simulink model "rfsoc_sdfec_model"  (R2020b)
settings: Solver=VariableStepAuto  StartTime=0.0  StopTime=T  RelTol=1e-3
values from neighbouring files (symbols this model uses):
  aximm_bit_count_reset = 0    [setup.m]
  aximm_bits = n_blocks * k    (= 80)    [setup.m]
  aximm_ctrl_word_dec = 0    [setup.m]
  aximm_ctrl_word_enc = 999    [setup.m]
  aximm_enable = 1    [setup.m]
  aximm_length = k * n_blocks    (= 80)    [setup.m]
  aximm_length_dec = n    (= 160)    [setup.m]
  aximm_length_enc = k/8    (= 10)    [setup.m]
  aximm_llr_scale = (1/noise_var) * llr_scale * 2    (= 200)    [setup.m]
  aximm_noise_std = sqrt(noise_var/2)    [setup.m]
  aximm_reset = 0    [setup.m]
  d = sqrt(-2*log([0:1/4095:1]))    [setup.m]
  fs = 100e6    (= 100000000)    [setup.m]
  generator_polynomial = '''z^13 + z^12 + z^11 + z^8 + 1'''    [setup.m]
libraries: hdlsllib x52, commseqgen3 x28, commblkcod2 x2, simulink x2
(part 1 of 2)
settings Model: Creator=ckb13136  LastModifiedBy=ckb13136
settings OptimizationCC: BlockReduction=off  ConditionallyExecuteInputs=off

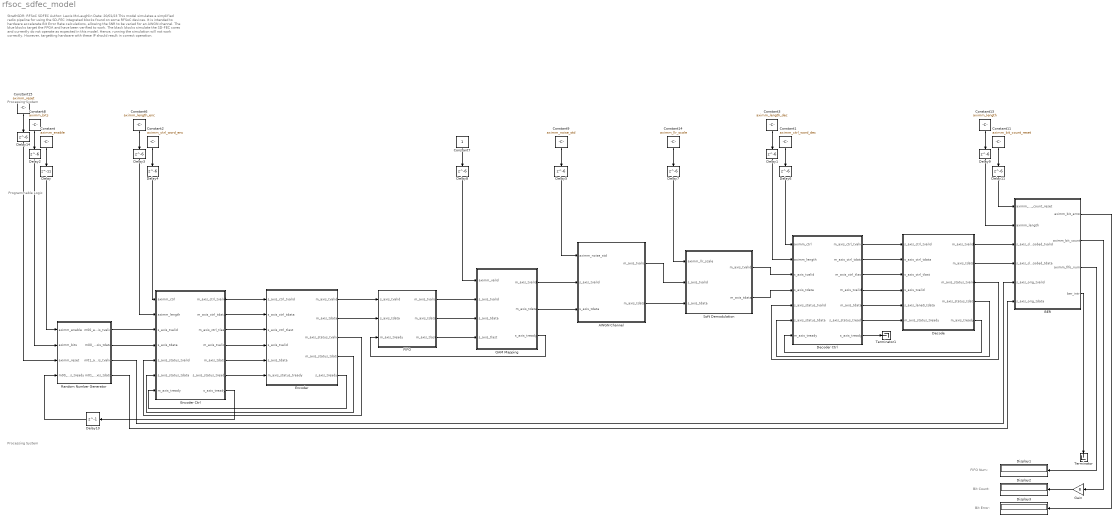
== system rfsoc_sdfec_model ==
  note: StrathSDR: RFSoC SDFEC
      | Author: Lewis McLaughlin
      | Date: 20/01/23
      |
      | This model simulates a simplified radio pipeline for using the SD-FEC integrated blocks found on some RFSoC devices. It is intended to hardware accelerate Bit Error Rate calculations, allowing the SNR to be varied for an AWGN channel. The blue blocks target the FPGA and have been verified to work. The black blocks simulate the SD-FEC cores and currently do not operate as expected in this model. Hence, running the simulation will not work correctly. However, targetting hardware with these IP should result in correct operation.
  note: FIFO Num:
  note: Programmable Logic
  note: Processing System
  note: Processing System
  note: Bit Count:
  note: Bit Error:
  AWGN Channel : Subsystem  TreatAsAtomicUnit=on
  BER : Subsystem  TreatAsAtomicUnit=on
  Constant : Constant  Value=aximm_enable  OutDataTypeStr=uint32  SampleTime=1/fs
  Constant1 : Constant  Value=aximm_ctrl_word_dec  OutDataTypeStr=uint32  SampleTime=1/fs
  Constant11 : Constant  Value=aximm_bit_count_reset  VectorParams1D=off  OutDataTypeStr=uint32  SampleTime=1/(fs)
  Constant13 : Constant  Value=aximm_length  OutDataTypeStr=uint32  SampleTime=1/(fs)
  Constant14 : Constant  Value=aximm_llr_scale  OutDataTypeStr=fixdt(0,32,12)  SampleTime=1/(fs)
  Constant15 : Constant  Value=aximm_reset  OutDataTypeStr=uint32  SampleTime=1/fs
  Constant2 : Constant  Value=aximm_ctrl_word_enc  OutDataTypeStr=uint32  SampleTime=1/fs
  Constant3 : Constant  Value=aximm_length_dec  OutDataTypeStr=uint32  SampleTime=1/fs
  Constant6 : Constant  Value=aximm_length_enc  OutDataTypeStr=uint32  SampleTime=1/fs
  Constant7 : Constant  OutDataTypeStr=uint32  SampleTime=1/fs
  Constant8 : Constant  Value=aximm_bits  OutDataTypeStr=uint32  SampleTime=1/fs
  Constant9 : Constant  Value=aximm_noise_std  OutDataTypeStr=fixdt(0,32,30)  SampleTime=1/(fs)
  Decode : Subsystem
  Decoder Ctrl : Subsystem  TreatAsAtomicUnit=on
  Delay : Delay  DelayLength=11
  Delay{1..9,11,14} (11 alike) : Delay  DelayLength=6
  Delay10 : Delay  DelayLength=1
  Display1 : Display
  Display2 : Display
  Display3 : Display
  Encoder : Subsystem
  Encoder Ctrl : Subsystem  TreatAsAtomicUnit=on
  FIFO : Subsystem
  Gain : Gain  Gain=8
  QAM Mapping : Subsystem  TreatAsAtomicUnit=on
  Random Number Generator : Subsystem  TreatAsAtomicUnit=on
  Soft Demodulation : Subsystem  TreatAsAtomicUnit=on
  Terminator : Terminator
  Terminator1 : Terminator
  wires:
  Delay/1 -> Random Number Generator/1(aximm_enable)
  Delay14/1 -> Random Number Generator/3(aximm_reset)
  Constant15/1 -> Delay14/1
  Delay2/1 -> Random Number Generator/2(aximm_bits)
  Constant/1 -> Delay/1
  Constant8/1 -> Delay2/1
  Random Number Generator/2(m00_axis_tdata) -> Encoder Ctrl/4(s_axis_tdata)
  Random Number Generator/1(m00_axis_tvalid) -> Encoder Ctrl/3(s_axis_tvalid)
  Encoder Ctrl/7(s_axis_tready) -> Delay10/1
  Encoder Ctrl/1(m_axis_ctrl_tvalid) -> Encoder/1(s_axis_ctrl_tvalid)
  Encoder Ctrl/2(m_axis_ctrl_tdata) -> Encoder/2(s_axis_ctrl_tdata)
  Encoder Ctrl/3(m_axis_ctrl_tlast) -> Encoder/3(s_axis_ctrl_tlast)
  Encoder Ctrl/4(m_axis_tvalid) -> Encoder/4(s_axis_tvalid)
  Encoder Ctrl/5(m_axis_tdata) -> Encoder/5(s_axis_tdata)
  Encoder Ctrl/6(s_axis_status_tready) -> Encoder/6(m_axis_status_tready)
  Encoder/4(m_axis_status_tdata) -> Encoder Ctrl/6(s_axis_status_tdata)
  Encoder/3(m_axis_status_tvalid) -> Encoder Ctrl/5(s_axis_status_tvalid)
  Delay4/1 -> Encoder Ctrl/1(aximm_ctrl)
  Constant2/1 -> Delay4/1
  Constant6/1 -> Delay3/1
  Delay3/1 -> Encoder Ctrl/2(aximm_length)
  Encoder/5(s_axis_tready) -> Encoder Ctrl/7(m_axis_tready)
  Encoder/1(m_axis_tvalid) -> FIFO/1(s_axis_tvalid)
  Encoder/2(m_axis_tdata) -> FIFO/2(s_axis_tdata)
  FIFO/1(m_axis_tvalid) -> QAM Mapping/2(s_axis_tvalid)
  FIFO/2(m_axis_tdata) -> QAM Mapping/3(s_axis_tdata)
  FIFO/3(m_axis_tlast) -> QAM Mapping/4(s_axis_tlast)
  QAM Mapping/3(s_axis_tready) -> FIFO/3(m_axis_tready)
  QAM Mapping/1(m_axis_tvalid) -> AWGN Channel/2(s_axis_tvalid)
  QAM Mapping/2(m_axis_tdata) -> AWGN Channel/3(s_axis_tdata)
  Constant9/1 -> Delay5/1
  Delay5/1 -> AWGN Channel/1(aximm_noise_std)
  AWGN Channel/2(m_axis_tdata) -> Soft Demodulation/3(s_axis_tdata)
  AWGN Channel/1(m_axis_tvalid) -> Soft Demodulation/2(s_axis_tvalid)
  Soft Demodulation/2(m_axis_tdata) -> Decoder Ctrl/4(s_axis_tdata)
  Soft Demodulation/1(m_axis_tvalid) -> Decoder Ctrl/3(s_axis_tvalid)
  Delay10/1 -> Random Number Generator/4(m00_axis_tready)
  Decoder Ctrl/1(m_axis_ctrl_tvalid) -> Decode/1(s_axis_ctrl_tvalid)
  Decoder Ctrl/2(m_axis_ctrl_tdata) -> Decode/2(s_axis_ctrl_tdata)
  Decoder Ctrl/3(m_axis_ctrl_tlast) -> Decode/3(s_axis_ctrl_tlast)
  Decoder Ctrl/4(m_axis_tvalid) -> Decode/4(s_axis_tvalid)
  Decoder Ctrl/5(m_axis_tdata) -> Decode/5(s_axis_lane0_tdata)
  Decoder Ctrl/6(s_axis_status_tready) -> Decode/6(m_axis_status_tready)
  Decode/5(m_axis_tready) -> Decoder Ctrl/7(m_axis_tready)
  Decode/4(m_axis_status_tdata) -> Decoder Ctrl/6(s_axis_status_tdata)
  Decode/3(m_axis_status_tvalid) -> Decoder Ctrl/5(s_axis_status_tvalid)
  Delay1/1 -> Decoder Ctrl/2(aximm_length)
  Constant3/1 -> Delay1/1
  Constant1/1 -> Delay6/1
  Delay6/1 -> Decoder Ctrl/1(aximm_ctrl)
  Constant14/1 -> Delay7/1
  Delay7/1 -> Soft Demodulation/1(aximm_llr_scale)
  Constant7/1 -> Delay8/1
  Delay8/1 -> QAM Mapping/1(aximm_valid)
  Decode/1(m_axis_tvalid) -> BER/3(s_axis_decoded_tvalid)
  Decode/2(m_axis_tdata) -> BER/4(s_axis_decoded_tdata)
  Random Number Generator/4(m01_axis_tdata) -> BER/6(s_axis_orig_tdata)
  Random Number Generator/3(m01_axis_tvalid) -> BER/5(s_axis_orig_tvalid)
  Delay11/1 -> BER/1(aximm_bit_count_reset)
  Constant11/1 -> Delay11/1
  Delay9/1 -> BER/2(aximm_length)
  Constant13/1 -> Delay9/1
  BER/4(ber_intr) -> Terminator/1
  BER/3(aximm_fifo_num) -> Display1/1
  BER/2(aximm_bit_count) -> Gain/1
  BER/1(aximm_bit_error) -> Display3/1
  Gain/1 -> Display2/1
  Decoder Ctrl/7(s_axis_tready) -> Terminator1/1

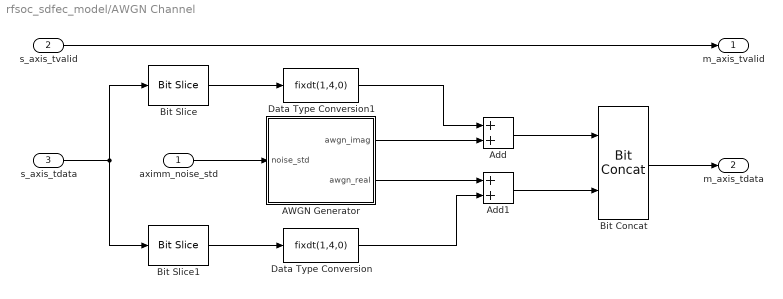
== system rfsoc_sdfec_model/AWGN Channel ==
  aximm_noise_std : Inport
  s_axis_tvalid : Inport  Port=2
  s_axis_tdata : Inport  Port=3
  AWGN Generator : Subsystem
  Add : Sum  OutDataTypeStr=fixdt(1,16,11)  SaturateOnIntegerOverflow=on
  Add1 : Sum  OutDataTypeStr=fixdt(1,16,11)  SaturateOnIntegerOverflow=on
  Bit Concat : hdlsllib/Logic and Bit Operations/Bit Concat  numInputs=2
  Bit Slice : hdlsllib/Logic and Bit Operations/Bit Slice  lidx=7  ridx=4
      settings: SourceProductBaseCode=SL
  Bit Slice1 : hdlsllib/Logic and Bit Operations/Bit Slice  lidx=3  ridx=0
      settings: SourceProductBaseCode=SL
  Data Type Conversion : DataTypeConversion  OutDataTypeStr=fixdt(1,4,0)  ConvertRealWorld=Stored Integer (SI)
  Data Type Conversion1 : DataTypeConversion  OutDataTypeStr=fixdt(1,4,0)  ConvertRealWorld=Stored Integer (SI)
  m_axis_tvalid : Outport
  m_axis_tdata : Outport  Port=2
  wires:
  Data Type Conversion1/1 -> Add/1
  Data Type Conversion/1 -> Add1/2
  Bit Slice/1 -> Data Type Conversion1/1
  Bit Slice1/1 -> Data Type Conversion/1
  s_axis_tvalid/1 -> m_axis_tvalid/1
  Bit Concat/1 -> m_axis_tdata/1
  s_axis_tdata/1 -> Bit Slice/1, Bit Slice1/1
  aximm_noise_std/1 -> AWGN Generator/1(noise_std)
  AWGN Generator/1(awgn_imag) -> Add/2
  AWGN Generator/2(awgn_real) -> Add1/1
  Add1/1 -> Bit Concat/2
  Add/1 -> Bit Concat/1

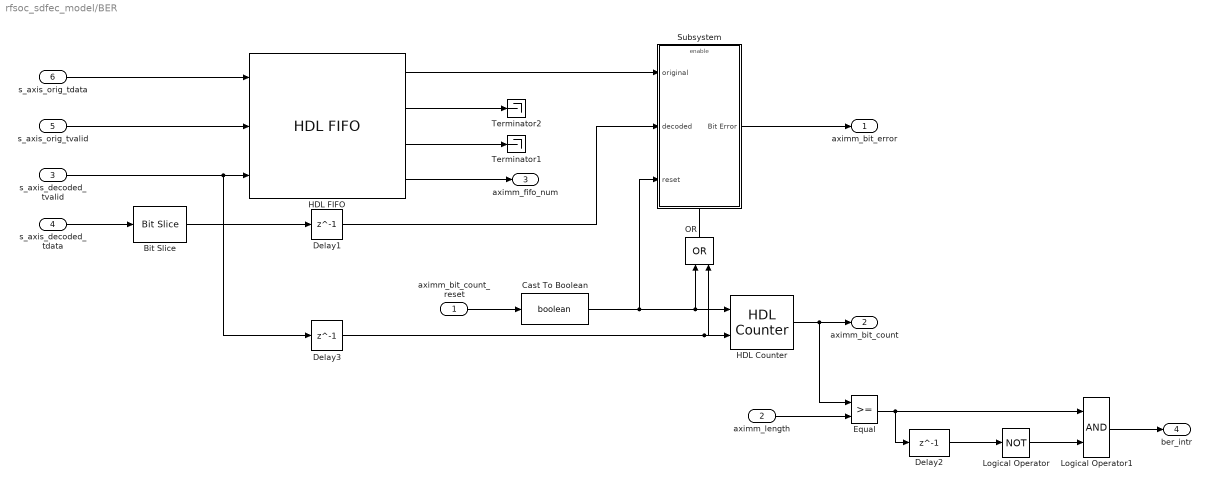
== system rfsoc_sdfec_model/BER ==
  aximm_bit_count_reset : Inport
  aximm_length : Inport  Port=2
  s_axis_decoded_tvalid : Inport  Port=3
  s_axis_decoded_tdata : Inport  Port=4
  s_axis_orig_tvalid : Inport  Port=5
  s_axis_orig_tdata : Inport  Port=6
  Bit Slice : hdlsllib/Logic and Bit Operations/Bit Slice  lidx=7  ridx=0
      settings: SourceProductBaseCode=SL
  Cast To Boolean : DataTypeConversion  OutDataTypeStr=boolean
  Delay1 : Delay  DelayLength=1
  Delay2 : Delay  DelayLength=1  InitialCondition=1  InputProcessing=Columns as channels (frame based)
  Delay3 : Delay  DelayLength=1
  Equal : RelationalOperator  OutDataTypeStr=boolean  RndMeth=Simplest
  HDL Counter : hdlsllib/Sources/HDL Counter  CountType=Free running  CountInit=0  CountStep=1  CountMax=25  CountFromType=Initial value  CountFrom=0  CountResetPort=on  CountLoadPort=off  CountEnbPort=on  CountDirPort=off  CountDataType=Unsigned  CountWordLen=32  CountFracLen=0  CountSampTime=1
  HDL FIFO : hdlsllib/HDL RAMs/HDL FIFO  fifo_size=65536  mode=Classic  ratio=1  push_msg=Warning  pop_msg=Warning  show_empty=on  show_full=on  show_num=on  LabelModeActiveChoice_Mode=Classic
      settings: SourceProductBaseCode=SL
  Logical Operator : Logic  Operator=NOT  Inputs=1
  Logical Operator1 : Logic
  OR : Logic  Operator=OR  IconShape=distinctive  AllPortsSameDT=off  OutDataTypeStr=boolean
  Subsystem : Subsystem
  Terminator1 : Terminator
  Terminator2 : Terminator
  aximm_bit_error : Outport
  aximm_bit_count : Outport  Port=2
  aximm_fifo_num : Outport  Port=3
  ber_intr : Outport  Port=4
  wires:
  HDL FIFO/4 -> aximm_fifo_num/1
  s_axis_decoded_tvalid/1 -> HDL FIFO/3, Delay3/1
  Delay3/1 -> OR/2, HDL Counter/2
  s_axis_decoded_tdata/1 -> Bit Slice/1
  s_axis_orig_tvalid/1 -> HDL FIFO/2
  HDL FIFO/3 -> Terminator1/1
  Subsystem/1(Bit Error) -> aximm_bit_error/1
  HDL FIFO/1 -> Subsystem/1(original)
  Delay1/1 -> Subsystem/2(decoded)
  HDL Counter/1 -> Equal/1, aximm_bit_count/1
  Bit Slice/1 -> Delay1/1
  s_axis_orig_tdata/1 -> HDL FIFO/1
  aximm_bit_count_reset/1 -> Cast To Boolean/1
  Cast To Boolean/1 -> OR/1, HDL Counter/1, Subsystem/3(reset)
  OR/1 -> Subsystem/Enable
  Logical Operator/1 -> Logical Operator1/2
  HDL FIFO/2 -> Terminator2/1
  Delay2/1 -> Logical Operator/1
  Logical Operator1/1 -> ber_intr/1
  Equal/1 -> Delay2/1, Logical Operator1/1
  aximm_length/1 -> Equal/2

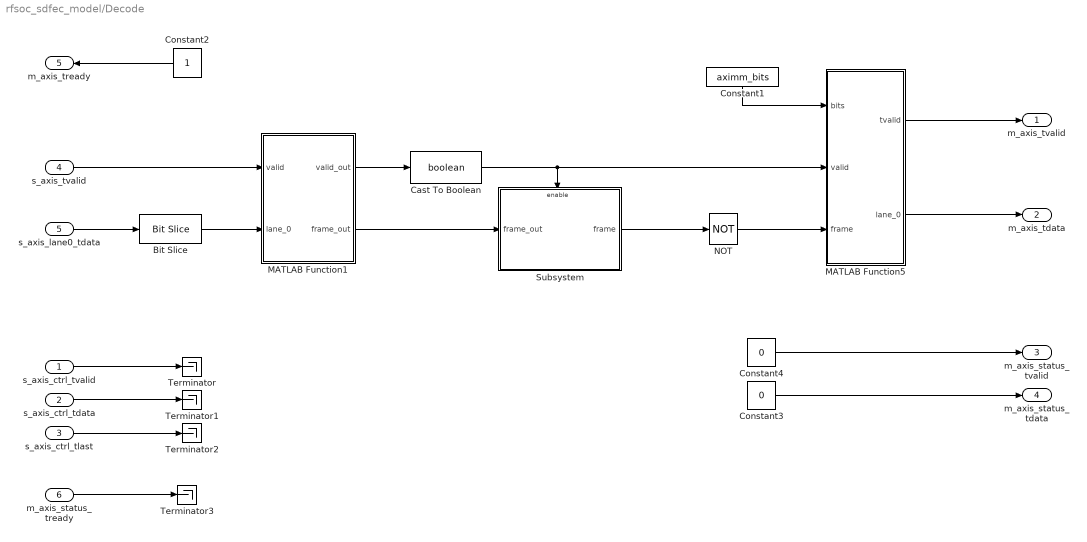
== system rfsoc_sdfec_model/Decode ==
  s_axis_ctrl_tvalid : Inport
  s_axis_ctrl_tdata : Inport  Port=2
  s_axis_ctrl_tlast : Inport  Port=3
  s_axis_tvalid : Inport  Port=4
  s_axis_lane0_tdata : Inport  Port=5
  m_axis_status_tready : Inport  Port=6
  Bit Slice : hdlsllib/Logic and Bit Operations/Bit Slice  lidx=31  ridx=0
      settings: SourceProductBaseCode=SL
  Cast To Boolean : DataTypeConversion  OutDataTypeStr=boolean
  Constant1 : Constant  Value=aximm_bits  OutDataTypeStr=uint32  SampleTime=1/fs
  Constant2 : Constant  OutDataTypeStr=boolean  SampleTime=1/fs
  Constant3 : Constant  Value=0  OutDataTypeStr=uint32  SampleTime=1/fs
  Constant4 : Constant  Value=0  OutDataTypeStr=boolean  SampleTime=1/fs
  MATLAB Function1 : MATLAB Function  TreatAsAtomicUnit=on
  MATLAB Function5 : MATLAB Function  TreatAsAtomicUnit=on
  NOT : Logic  Operator=NOT  IconShape=distinctive  AllPortsSameDT=off  OutDataTypeStr=boolean
  Subsystem : Subsystem
  Terminator{,1..3} (4 alike) : Terminator
  m_axis_tvalid : Outport
  m_axis_tdata : Outport  Port=2
  m_axis_status_tvalid : Outport  Port=3
  m_axis_status_tdata : Outport  Port=4
  m_axis_tready : Outport  Port=5
  wires:
  MATLAB Function5/1(tvalid) -> m_axis_tvalid/1
  Cast To Boolean/1 -> Subsystem/Enable, MATLAB Function5/2(valid)
  MATLAB Function5/2(lane_0) -> m_axis_tdata/1
  Constant1/1 -> MATLAB Function5/1(bits)
  s_axis_lane0_tdata/1 -> Bit Slice/1
  MATLAB Function1/1(valid_out) -> Cast To Boolean/1
  s_axis_tvalid/1 -> MATLAB Function1/1(valid)
  Subsystem/1(frame) -> NOT/1
  Constant3/1 -> m_axis_status_tdata/1
  Constant4/1 -> m_axis_status_tvalid/1
  m_axis_status_tready/1 -> Terminator3/1
  s_axis_ctrl_tlast/1 -> Terminator2/1
  s_axis_ctrl_tdata/1 -> Terminator1/1
  s_axis_ctrl_tvalid/1 -> Terminator/1
  Constant2/1 -> m_axis_tready/1
  MATLAB Function1/2(frame_out) -> Subsystem/1(frame_out)
  Bit Slice/1 -> MATLAB Function1/2(lane_0)
  NOT/1 -> MATLAB Function5/3(frame)

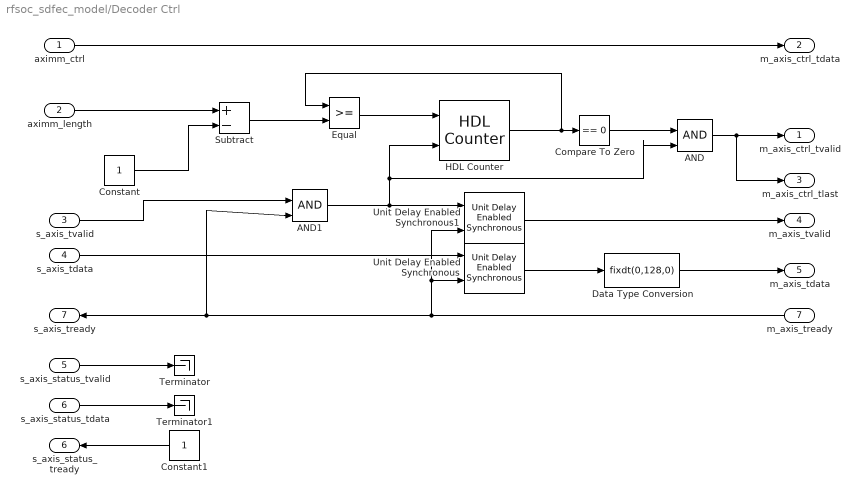
== system rfsoc_sdfec_model/Decoder Ctrl ==
  aximm_ctrl : Inport
  aximm_length : Inport  Port=2
  s_axis_tvalid : Inport  Port=3
  s_axis_tdata : Inport  Port=4
  s_axis_status_tvalid : Inport  Port=5
  s_axis_status_tdata : Inport  Port=6
  m_axis_tready : Inport  Port=7
  AND : Logic  IconShape=distinctive  AllPortsSameDT=off  OutDataTypeStr=boolean
  AND1 : Logic  IconShape=distinctive  AllPortsSameDT=off  OutDataTypeStr=boolean
  Compare To Zero : simulink/Logic and Bit Operations/Compare To Zero  relop===  OutDataTypeStr=boolean
  Constant : Constant  OutDataTypeStr=uint8  SampleTime=-1
  Constant1 : Constant  OutDataTypeStr=boolean  SampleTime=-1
  Data Type Conversion : DataTypeConversion  OutDataTypeStr=fixdt(0,128,0)
  Equal : RelationalOperator  OutDataTypeStr=boolean  RndMeth=Simplest
  HDL Counter : hdlsllib/Sources/HDL Counter  CountType=Free running  CountInit=0  CountStep=1  CountMax=2^32 - 1  CountFromType=Initial value  CountFrom=0  CountResetPort=on  CountLoadPort=off  CountEnbPort=on  CountDirPort=off  CountDataType=Unsigned  CountWordLen=32  CountFracLen=0  CountSampTime=1
  Subtract : Sum  Inputs=+-
  Terminator : Terminator
  Terminator1 : Terminator
  Unit Delay Enabled Synchronous : hdlsllib/Discrete/Unit Delay Enabled Synchronous  InitialCondition=0.0  SampleTime=-1
      settings: SourceProductBaseCode=SL
  Unit Delay Enabled Synchronous1 : hdlsllib/Discrete/Unit Delay Enabled Synchronous  InitialCondition=0.0  SampleTime=-1
      settings: SourceProductBaseCode=SL
  m_axis_ctrl_tvalid : Outport
  m_axis_ctrl_tdata : Outport  Port=2
  m_axis_ctrl_tlast : Outport  Port=3
  m_axis_tvalid : Outport  Port=4
  m_axis_tdata : Outport  Port=5
  s_axis_status_tready : Outport  Port=6
  s_axis_tready : Outport  Port=7
  wires:
  Equal/1 -> HDL Counter/1
  Subtract/1 -> Equal/2
  aximm_ctrl/1 -> m_axis_ctrl_tdata/1
  HDL Counter/1 -> Compare To Zero/1, Equal/1
  AND1/1 -> Unit Delay Enabled Synchronous1/1, HDL Counter/2, AND/2
  s_axis_tdata/1 -> Unit Delay Enabled Synchronous/1
  Unit Delay Enabled Synchronous1/1 -> m_axis_tvalid/1
  Unit Delay Enabled Synchronous/1 -> Data Type Conversion/1
  Compare To Zero/1 -> AND/1
  AND/1 -> m_axis_ctrl_tlast/1, m_axis_ctrl_tvalid/1
  aximm_length/1 -> Subtract/1
  Constant/1 -> Subtract/2
  Constant1/1 -> s_axis_status_tready/1
  s_axis_status_tvalid/1 -> Terminator/1
  s_axis_status_tdata/1 -> Terminator1/1
  Data Type Conversion/1 -> m_axis_tdata/1
  m_axis_tready/1 -> Unit Delay Enabled Synchronous1/2, Unit Delay Enabled Synchronous/2, AND1/2, s_axis_tready/1
  s_axis_tvalid/1 -> AND1/1

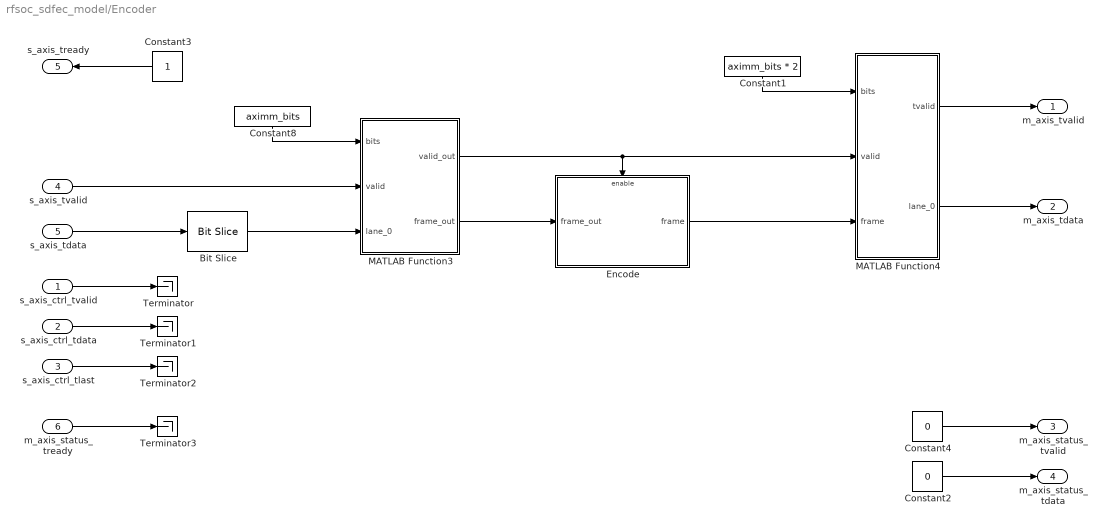
== system rfsoc_sdfec_model/Encoder ==
  s_axis_ctrl_tvalid : Inport
  s_axis_ctrl_tdata : Inport  Port=2
  s_axis_ctrl_tlast : Inport  Port=3
  s_axis_tvalid : Inport  Port=4
  s_axis_tdata : Inport  Port=5
  m_axis_status_tready : Inport  Port=6
  Bit Slice : hdlsllib/Logic and Bit Operations/Bit Slice  lidx=7  ridx=0
      settings: SourceProductBaseCode=SL
  Constant1 : Constant  Value=aximm_bits * 2  OutDataTypeStr=uint32  SampleTime=1/(fs)
  Constant2 : Constant  Value=0  OutDataTypeStr=uint32  SampleTime=1/fs
  Constant3 : Constant  OutDataTypeStr=boolean  SampleTime=1/fs
  Constant4 : Constant  Value=0  OutDataTypeStr=boolean  SampleTime=1/fs
  Constant8 : Constant  Value=aximm_bits  OutDataTypeStr=uint32  SampleTime=1/(fs)
  Encode : Subsystem
  MATLAB Function3 : MATLAB Function  TreatAsAtomicUnit=on
  MATLAB Function4 : MATLAB Function  TreatAsAtomicUnit=on
  Terminator{,1..3} (4 alike) : Terminator
  m_axis_tvalid : Outport
  m_axis_tdata : Outport  Port=2
  m_axis_status_tvalid : Outport  Port=3
  m_axis_status_tdata : Outport  Port=4
  s_axis_tready : Outport  Port=5
  wires:
  Constant4/1 -> m_axis_status_tvalid/1
  s_axis_ctrl_tvalid/1 -> Terminator/1
  s_axis_ctrl_tdata/1 -> Terminator1/1
  s_axis_ctrl_tlast/1 -> Terminator2/1
  m_axis_status_tready/1 -> Terminator3/1
  MATLAB Function3/2(frame_out) -> Encode/1(frame_out)
  s_axis_tvalid/1 -> MATLAB Function3/2(valid)
  s_axis_tdata/1 -> Bit Slice/1
  Constant8/1 -> MATLAB Function3/1(bits)
  Encode/1(frame) -> MATLAB Function4/3(frame)
  MATLAB Function4/1(tvalid) -> m_axis_tvalid/1
  Constant1/1 -> MATLAB Function4/1(bits)
  MATLAB Function4/2(lane_0) -> m_axis_tdata/1
  Constant2/1 -> m_axis_status_tdata/1
  MATLAB Function3/1(valid_out) -> Encode/Enable, MATLAB Function4/2(valid)
  Bit Slice/1 -> MATLAB Function3/3(lane_0)
  Constant3/1 -> s_axis_tready/1

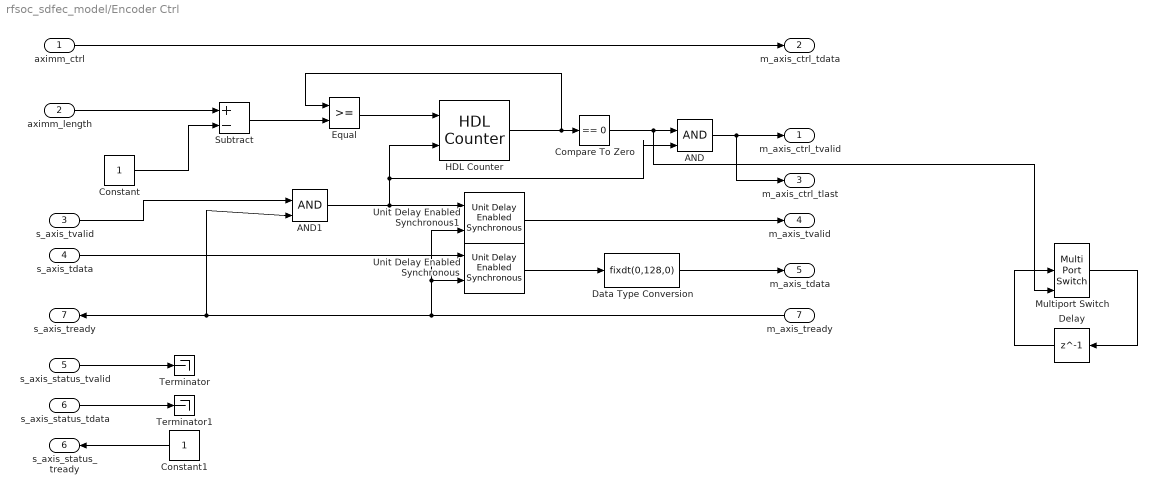
== system rfsoc_sdfec_model/Encoder Ctrl ==
  aximm_ctrl : Inport
  aximm_length : Inport  Port=2
  s_axis_tvalid : Inport  Port=3
  s_axis_tdata : Inport  Port=4
  s_axis_status_tvalid : Inport  Port=5
  s_axis_status_tdata : Inport  Port=6
  m_axis_tready : Inport  Port=7
  AND : Logic  IconShape=distinctive  AllPortsSameDT=off  OutDataTypeStr=boolean
  AND1 : Logic  IconShape=distinctive  AllPortsSameDT=off  OutDataTypeStr=boolean
  Compare To Zero : simulink/Logic and Bit Operations/Compare To Zero  relop===  OutDataTypeStr=boolean
  Constant : Constant  OutDataTypeStr=uint8  SampleTime=-1
  Constant1 : Constant  OutDataTypeStr=boolean  SampleTime=-1
  Data Type Conversion : DataTypeConversion  OutDataTypeStr=fixdt(0,128,0)
  Delay : Delay  DelayLength=1
  Equal : RelationalOperator  OutDataTypeStr=boolean  RndMeth=Simplest
  HDL Counter : hdlsllib/Sources/HDL Counter  CountType=Free running  CountInit=0  CountStep=1  CountMax=2^32 - 1  CountFromType=Initial value  CountFrom=0  CountResetPort=on  CountLoadPort=off  CountEnbPort=on  CountDirPort=off  CountDataType=Unsigned  CountWordLen=32  CountFracLen=0  CountSampTime=1
  Multiport Switch : MultiPortSwitch  DataPortOrder=Zero-based contiguous  Inputs=2  zeroidx=on
  Subtract : Sum  Inputs=+-
  Terminator : Terminator
  Terminator1 : Terminator
  Unit Delay Enabled Synchronous : hdlsllib/Discrete/Unit Delay Enabled Synchronous  InitialCondition=0.0  SampleTime=-1
      settings: SourceProductBaseCode=SL
  Unit Delay Enabled Synchronous1 : hdlsllib/Discrete/Unit Delay Enabled Synchronous  InitialCondition=0.0  SampleTime=-1
      settings: SourceProductBaseCode=SL
  m_axis_ctrl_tvalid : Outport
  m_axis_ctrl_tdata : Outport  Port=2
  m_axis_ctrl_tlast : Outport  Port=3
  m_axis_tvalid : Outport  Port=4
  m_axis_tdata : Outport  Port=5
  s_axis_status_tready : Outport  Port=6
  s_axis_tready : Outport  Port=7
  wires:
  s_axis_tvalid/1 -> AND1/1
  m_axis_tready/1 -> s_axis_tready/1, AND1/2, Unit Delay Enabled Synchronous/2, Unit Delay Enabled Synchronous1/2
  Data Type Conversion/1 -> m_axis_tdata/1
  s_axis_status_tdata/1 -> Terminator1/1
  s_axis_status_tvalid/1 -> Terminator/1
  Constant1/1 -> s_axis_status_tready/1
  Constant/1 -> Subtract/2
  aximm_length/1 -> Subtract/1
  AND/1 -> m_axis_ctrl_tvalid/1, m_axis_ctrl_tlast/1
  Compare To Zero/1 -> Multiport Switch/3, AND/1
  Unit Delay Enabled Synchronous/1 -> Data Type Conversion/1
  Unit Delay Enabled Synchronous1/1 -> m_axis_tvalid/1
  s_axis_tdata/1 -> Unit Delay Enabled Synchronous/1
  AND1/1 -> AND/2, HDL Counter/2, Unit Delay Enabled Synchronous1/1
  HDL Counter/1 -> Equal/1, Compare To Zero/1
  aximm_ctrl/1 -> m_axis_ctrl_tdata/1
  Subtract/1 -> Equal/2
  Equal/1 -> HDL Counter/1
  Multiport Switch/1 -> Delay/1
  Delay/1 -> Multiport Switch/2

== system rfsoc_sdfec_model/FIFO ==
  s_axis_tvalid : Inport
  s_axis_tdata : Inport  Port=2
  m_axis_tready : Inport  Port=3
  AND1 : Logic  IconShape=distinctive  AllPortsSameDT=off  OutDataTypeStr=boolean
  AND2 : Logic  IconShape=distinctive  AllPortsSameDT=off  OutDataTypeStr=boolean
  Constant : Constant  Value=0  OutDataTypeStr=boolean  SampleTime=1/fs
  HDL FIFO : hdlsllib/HDL RAMs/HDL FIFO  fifo_size=2048  mode=FWFT  ratio=1  push_msg=Warning  pop_msg=Warning  show_empty=on  show_full=on  show_num=on  LabelModeActiveChoice_Mode=FWFT
      settings: SourceProductBaseCode=SL
  NOT1 : Logic  Operator=NOT  IconShape=distinctive  AllPortsSameDT=off  OutDataTypeStr=boolean
  NOT3 : Logic  Operator=NOT  IconShape=distinctive  AllPortsSameDT=off  OutDataTypeStr=boolean
  m_axis_tvalid : Outport
  m_axis_tdata : Outport  Port=2
  m_axis_tlast : Outport  Port=3
  wires:
  AND1/1 -> HDL FIFO/3
  HDL FIFO/3 -> NOT3/1
  AND2/1 -> HDL FIFO/2
  HDL FIFO/2 -> NOT1/1
  m_axis_tready/1 -> AND1/2
  HDL FIFO/1 -> m_axis_tdata/1
  NOT1/1 -> m_axis_tvalid/1, AND1/1  "tvalid"
  NOT3/1 -> AND2/2  "tvalid"
  s_axis_tvalid/1 -> AND2/1
  s_axis_tdata/1 -> HDL FIFO/1
  Constant/1 -> m_axis_tlast/1

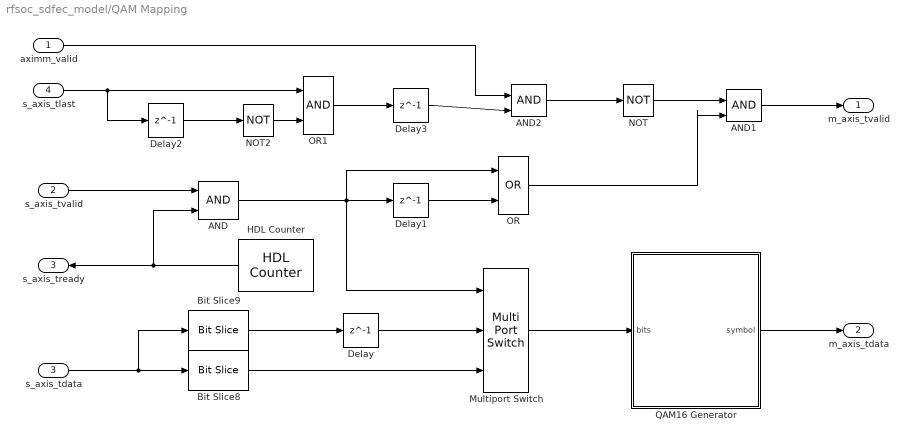
== system rfsoc_sdfec_model/QAM Mapping ==
  aximm_valid : Inport
  s_axis_tvalid : Inport  Port=2
  s_axis_tdata : Inport  Port=3
  s_axis_tlast : Inport  Port=4
  AND : Logic  IconShape=distinctive  AllPortsSameDT=off  OutDataTypeStr=boolean
  AND1 : Logic  IconShape=distinctive  AllPortsSameDT=off  OutDataTypeStr=boolean
  AND2 : Logic  IconShape=distinctive  AllPortsSameDT=off  OutDataTypeStr=boolean
  Bit Slice8 : hdlsllib/Logic and Bit Operations/Bit Slice  lidx=3  ridx=0
      settings: SourceProductBaseCode=SL
  Bit Slice9 : hdlsllib/Logic and Bit Operations/Bit Slice  lidx=7  ridx=4
      settings: SourceProductBaseCode=SL
  Delay{,1..3} (4 alike) : Delay  DelayLength=1
  HDL Counter : hdlsllib/Sources/HDL Counter  CountType=Count limited  CountInit=0  CountStep=1  CountMax=1  CountFromType=Initial value  CountFrom=0  CountResetPort=off  CountLoadPort=off  CountEnbPort=off  CountDirPort=off  CountDataType=Unsigned  CountWordLen=1  CountFracLen=0  CountSampTime=1/fs
  Multiport Switch : MultiPortSwitch  DataPortOrder=Zero-based contiguous  Inputs=2  zeroidx=on
  NOT : Logic  Operator=NOT  IconShape=distinctive  AllPortsSameDT=off  OutDataTypeStr=boolean
  NOT2 : Logic  Operator=NOT  IconShape=distinctive  AllPortsSameDT=off  OutDataTypeStr=boolean
  OR : Logic  Operator=OR  IconShape=distinctive  AllPortsSameDT=off  OutDataTypeStr=boolean
  OR1 : Logic  IconShape=distinctive  AllPortsSameDT=off  OutDataTypeStr=boolean
  QAM16 Generator : Subsystem
  m_axis_tvalid : Outport
  m_axis_tdata : Outport  Port=2
  s_axis_tready : Outport  Port=3
  wires:
  NOT2/1 -> OR1/2
  s_axis_tlast/1 -> Delay2/1, OR1/1
  NOT/1 -> AND1/1
  AND2/1 -> NOT/1
  Delay3/1 -> AND2/2
  OR1/1 -> Delay3/1
  Delay2/1 -> NOT2/1
  Multiport Switch/1 -> QAM16 Generator/1(bits)
  AND1/1 -> m_axis_tvalid/1
  Delay1/1 -> OR/2
  OR/1 -> AND1/2
  aximm_valid/1 -> AND2/1
  AND/1 -> Multiport Switch/1, Delay1/1, OR/1
  QAM16 Generator/1(symbol) -> m_axis_tdata/1
  HDL Counter/1 -> s_axis_tready/1, AND/2
  Delay/1 -> Multiport Switch/2
  s_axis_tvalid/1 -> AND/1
  Bit Slice8/1 -> Multiport Switch/3
  Bit Slice9/1 -> Delay/1
  s_axis_tdata/1 -> Bit Slice9/1, Bit Slice8/1

== system rfsoc_sdfec_model/Random Number Generator ==
  aximm_enable : Inport
  aximm_bits : Inport  Port=2
  aximm_reset : Inport  Port=3
  m00_axis_tready : Inport  Port=4
  AND : Logic  IconShape=distinctive  AllPortsSameDT=off  OutDataTypeStr=boolean
  Cast To Boolean1 : DataTypeConversion  OutDataTypeStr=boolean
  Random Number Generator : Subsystem  mask{bits=8, gen_poly=generator_polynomial}
      mask prompts: bits "Data Bits:"; gen_poly "Generator Polynomial:"
      mask init:
      | random_gen = gcb;
      | 
      | %set_param(random_gen, 'LinkStatus', 'none');
      | 
      | block_handles = Simulink.findBlocks(gcb);
      | block_names = getfullname(block_handles);
      | 
      | out_block = sprintf('%s/data', random_gen);
      | in_block = sprintf('%s/reset', random_gen);
      | enable_block = sprintf('%s/enable', random_gen);
      | 
      | keep_blocks = {out_block, in_block, enable_block};
      | 
      | for i = 1:length(block_names)
      |     if ~ismember(block_names{i}, keep_blocks)
      |         delete_block(block_names{i});
      |     end
      | end
      | delete_line(find_system(random_gen,'LookUnderMasks', 'all','FindAll','on','type','line'));
      | 
      | % Add all PN Sequence Generators 
      | for bit = 1:bits
      |     current_block = sprintf('%s/bit%d', random_gen, bit-1);
      |     add_block('commseqgen3/PN Sequence Generator', current_block);
      |     position = get_param(current_block, 'position');
      |     if bit == 1
      |         start_position = position;
      |     end
      |     new_position = position + ([0 60 0 60] * (bit-1));
      |     set_param(current_block, 'position', new_position);
      |     set_param(current_block, 'outDataType', 'boolean');
      |     set_param(current_block, 'reset', 'on');
      |     set_param(current_block, 'Ts', '-1');
      |     set_param(current_block, 'poly', gen_poly);
      |     
      |     val = dec2bin(randi(2^13 - 1), 13);
      |     str = '[';
      |     for i = 1:13
      |         str(end+1:end+2) = [' ' (val(i))];
      |     end
      |     str(end+1) = ']';
      |     set_param(current_block, 'ini_sta', str);
      | end
      | 
      | % Add the Bit Concat
      | concat_block = sprintf('%s/concat', random_gen);
      | add_block('hdlsllib/Logic and Bit Operations/Bit Concat', concat_block);
      | set_param(concat_block, 'numInputs', num2str(bits));
      | position = new_position + [150 0 150 0];
      | position(2) = start_position(2);
      | set_param(concat_block, 'position', position);
      | 
      | % Add Input and Outputs
      | out_position = get_param(out_block, 'position');
      | height = out_position(4) - out_position(2);
      | width = out_position(3) - out_position(1);
      | middle_h = (position(4) - position(2))/2 + position(2);
      | out_position = [position(1) + 150, middle_h - height/2, position(1) + 150 + width, middle_h + height/2];
      | set_param(out_block, 'position', out_position);
      | 
      | in_position = [position(1) - 300, middle_h - height/2, position(1) - 300 + width, middle_h + height/2];
      | set_param(in_block, 'position', in_position);
      | 
      | % enable_position = get_param(in_position, 'position');
      | set_param(enable_block, 'position', in_position - [0 100 0 100]);
      | 
      | % Connect Ports
      | for bit = 1:bits
      |     add_line(random_gen,'reset/1', sprintf('bit%d/1', bit-1));
      |     add_line(random_gen,sprintf('bit%d/1', bit-1), sprintf('concat/%d', bit));
      | end
      | add_line(random_gen,'concat/1','data/1');
      mask DialogControl DescGroupVar Prompt: N-Bit Random Number Generator
      mask DialogControl DescTextVar Prompt: This block will create a n-bit random number generator. Provide a polynomial and the number of bits. Information on polynomials for maximal LFSRs can be found:  https://en.wikipedia.org/wiki/Linear-feedback_shift_register For example: ''z^13 + z^12 + z^11 + z^8 + 1''
  rising_edge : Subsystem
  tvalid hold : Subsystem
  m00_axis_tvalid : Outport
  m00_axis_tdata : Outport  Port=2
  m01_axis_tvalid : Outport  Port=3
  m01_axis_tdata : Outport  Port=4
  wires:
  Random Number Generator/1(data) -> m01_axis_tdata/1, m00_axis_tdata/1
  tvalid hold/1(enable) -> AND/2
  Cast To Boolean1/1 -> Random Number Generator/1(reset)
  aximm_bits/1 -> tvalid hold/3(comparator)
  rising_edge/1(pulse) -> tvalid hold/2(trigger)
  aximm_enable/1 -> rising_edge/1(in)
  aximm_reset/1 -> Cast To Boolean1/1
  m00_axis_tready/1 -> tvalid hold/1(en), AND/1
  AND/1 -> Random Number Generator/Enable, m01_axis_tvalid/1, m00_axis_tvalid/1

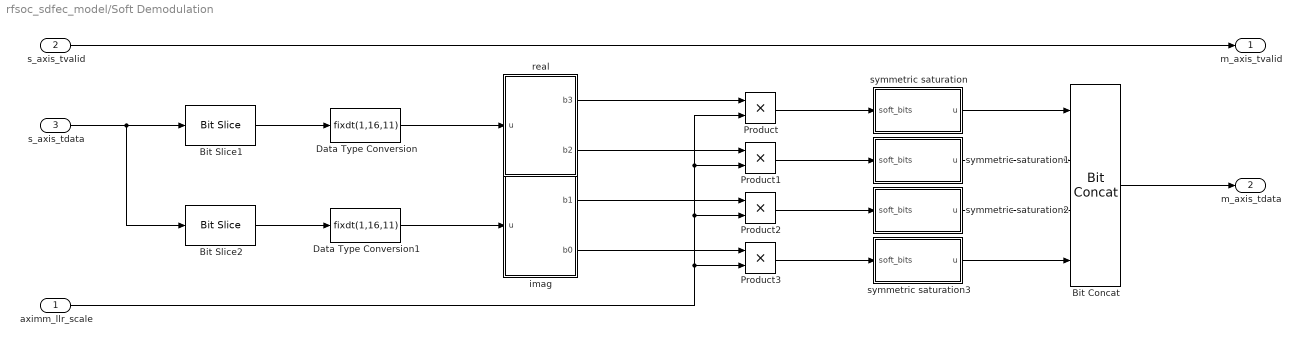
== system rfsoc_sdfec_model/Soft Demodulation ==
  aximm_llr_scale : Inport
  s_axis_tvalid : Inport  Port=2
  s_axis_tdata : Inport  Port=3
  Bit Concat : hdlsllib/Logic and Bit Operations/Bit Concat  numInputs=4
  Bit Slice1 : hdlsllib/Logic and Bit Operations/Bit Slice  lidx=15  ridx=0
      settings: SourceProductBaseCode=SL
  Bit Slice2 : hdlsllib/Logic and Bit Operations/Bit Slice  lidx=31  ridx=16
      settings: SourceProductBaseCode=SL
  Data Type Conversion : DataTypeConversion  OutDataTypeStr=fixdt(1,16,11)  ConvertRealWorld=Stored Integer (SI)
  Data Type Conversion1 : DataTypeConversion  OutDataTypeStr=fixdt(1,16,11)  ConvertRealWorld=Stored Integer (SI)
  Product{,1..3} (4 alike) : Product  OutDataTypeStr=fixdt(1,6,2)  SaturateOnIntegerOverflow=on
  imag : MATLAB Function  TreatAsAtomicUnit=on
  real : MATLAB Function  TreatAsAtomicUnit=on
  symmetric saturation : Subsystem
  symmetric saturation1 : Subsystem
  symmetric saturation2 : Subsystem
  symmetric saturation3 : Subsystem
  m_axis_tvalid : Outport
  m_axis_tdata : Outport  Port=2
  wires:
  Product/1 -> symmetric saturation/1(soft_bits)
  Data Type Conversion1/1 -> imag/1(u)
  Data Type Conversion/1 -> real/1(u)
  Bit Slice2/1 -> Data Type Conversion1/1
  Bit Slice1/1 -> Data Type Conversion/1
  s_axis_tvalid/1 -> m_axis_tvalid/1
  s_axis_tdata/1 -> Bit Slice2/1, Bit Slice1/1
  real/1(b3) -> Product/1
  real/2(b2) -> Product1/1
  imag/2(b0) -> Product3/1
  aximm_llr_scale/1 -> Product/2, Product1/2, Product2/2, Product3/2
  imag/1(b1) -> Product2/1
  Product1/1 -> symmetric saturation1/1(soft_bits)
  Product2/1 -> symmetric saturation2/1(soft_bits)
  Product3/1 -> symmetric saturation3/1(soft_bits)
  symmetric saturation/1(u) -> Bit Concat/1
  symmetric saturation1/1(u) -> Bit Concat/2
  symmetric saturation2/1(u) -> Bit Concat/3
  symmetric saturation3/1(u) -> Bit Concat/4
  Bit Concat/1 -> m_axis_tdata/1

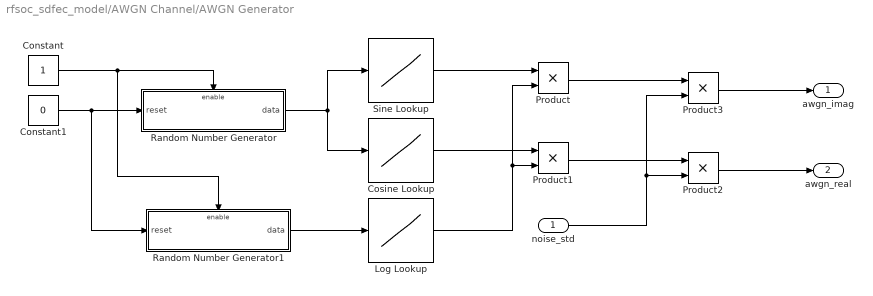
== system rfsoc_sdfec_model/AWGN Channel/AWGN Generator ==
  noise_std : Inport
  Constant : Constant  OutDataTypeStr=boolean  SampleTime=1/fs
  Constant1 : Constant  Value=0  OutDataTypeStr=boolean  SampleTime=1/fs
  Cosine Lookup : Lookup_n-D  NumberOfTableDimensions=1  BreakpointsForDimension1=[0:255]  IndexSearchMethod=Evenly spaced points  Table=cos([0:255]*2*pi/256)  InterpMethod=Flat  ExtrapMethod=Clip  DiagnosticForOutOfRangeInput=Error  UseLastTableValue=on  OutDataTypeStr=fixdt(1,16,14)  RndMeth=Simplest  InputSameDT=on
  Log Lookup : Lookup_n-D  NumberOfTableDimensions=1  BreakpointsForDimension1=[0:4095]  BreakpointsForDimension1DataTypeStr=fixdt(0,12,0)  IndexSearchMethod=Evenly spaced points  Table=d  InterpMethod=Flat  ExtrapMethod=Clip  DiagnosticForOutOfRangeInput=Error  InternalRulePriority=Speed  OutDataTypeStr=fixdt(1,17,13)  RndMeth=Simplest  InputSameDT=on
  Product : Product  OutDataTypeStr=fixdt(1,17,13)  RndMeth=Round  SaturateOnIntegerOverflow=on
  Product1 : Product  OutDataTypeStr=fixdt(1,17,13)  RndMeth=Round  SaturateOnIntegerOverflow=on
  Product2 : Product  OutDataTypeStr=fixdt(1,18,14)  RndMeth=Round
  Product3 : Product  OutDataTypeStr=fixdt(1,18,14)  RndMeth=Round
  Random Number Generator : Subsystem  mask{bits=8, gen_poly=generator_polynomial}
      mask prompts: bits "Data Bits:"; gen_poly "Generator Polynomial:"
      mask init:
      | % random_gen = gcb;
      | % 
      | % %set_param(random_gen, 'LinkStatus', 'none');
      | % 
      | % block_handles = Simulink.findBlocks(gcb);
      | % block_names = getfullname(block_handles);
      | % 
      | % out_block = sprintf('%s/data', random_gen);
      | % in_block = sprintf('%s/reset', random_gen);
      | % enable_block = sprintf('%s/enable', random_gen);
      | % 
      | % keep_blocks = {out_block, in_block, enable_block};
      | % 
      | % for i = 1:length(block_names)
      | %     if ~ismember(block_names{i}, keep_blocks)
      | %         delete_block(block_names{i});
      | %     end
      | % end
      | % delete_line(find_system(random_gen,'LookUnderMasks', 'all','FindAll','on','type','line'));
      | % 
      | % % Add all PN Sequence Generators 
      | % for bit = 1:bits
      | %     current_block = sprintf('%s/bit%d', random_gen, bit-1);
      | %     add_block('commseqgen3/PN Sequence Generator', current_block);
      | %     position = get_param(current_block, 'position');
      | %     if bit == 1
      | %         start_position = position;
      | %     end
      | %     new_position = position + ([0 60 0 60] * (bit-1));
      | %     set_param(current_block, 'position', new_position);
      | %     set_param(current_block, 'outDataType', 'boolean');
      | %     set_param(current_block, 'reset', 'on');
      | %     set_param(current_block, 'Ts', '-1');
      | %     set_param(current_block, 'poly', gen_poly);
      | %     
      | %     val = dec2bin(randi(2^13 - 1), 13);
      | %     str = '[';
      | %     for i = 1:13
      | %         str(end+1:end+2) = [' ' (val(i))];
      | %     end
      | %     str(end+1) = ']';
      | %     set_param(current_block, 'ini_sta', str);
      | % end
      | % 
      | % % Add the Bit Concat
      | % concat_block = sprintf('%s/concat', random_gen);
      | % add_block('hdlsllib/Logic and Bit Operations/Bit Concat', concat_block);
      | % set_param(concat_block, 'numInputs', num2str(bits));
      | % position = new_position + [150 0 150 0];
      | % position(2) = start_position(2);
      | % set_param(concat_block, 'position', position);
      | % 
      | % % Add Input and Outputs
      | % out_position = get_param(out_block, 'position');
      | % height = out_position(4) - out_position(2);
      | % width = out_position(3) - out_position(1);
      | % middle_h = (position(4) - position(2))/2 + position(2);
      | % out_position = [position(1) + 150, middle_h - height/2, position(1) + 150 + width, middle_h + height/2];
      | % set_param(out_block, 'position', out_position);
      | % 
      | % in_position = [position(1) - 300, middle_h - height/2, position(1) - 300 + width, middle_h + height/2];
      | % set_param(in_block, 'position', in_position);
      | % 
      | % % enable_position = get_param(in_position, 'position');
      | % set_param(enable_block, 'position', in_position - [0 100 0 100]);
      | % 
      | % % Connect Ports
      | % for bit = 1:bits
      | %     add_line(random_gen,'reset/1', sprintf('bit%d/1', bit-1));
      | %     add_line(random_gen,sprintf('bit%d/1', bit-1), sprintf('concat/%d', bit));
      | % end
      | % add_line(random_gen,'concat/1','data/1');
      mask DialogControl DescGroupVar Prompt: N-Bit Random Number Generator
      mask DialogControl DescTextVar Prompt: This block will create a n-bit random number generator. Provide a polynomial and the number of bits. Information on polynomials for maximal LFSRs can be found:  https://en.wikipedia.org/wiki/Linear-feedback_shift_register For example: ''z^13 + z^12 + z^11 + z^8 + 1''
  Random Number Generator1 : Subsystem  mask{bits=12, gen_poly=generator_polynomial}
      mask prompts: bits "Data Bits:"; gen_poly "Generator Polynomial:"
      mask init: same as rfsoc_sdfec_model/AWGN Channel/AWGN Generator/Random Number Generator
      mask DialogControl DescGroupVar Prompt: N-Bit Random Number Generator
      mask DialogControl DescTextVar Prompt: This block will create a n-bit random number generator. Provide a polynomial and the number of bits. Information on polynomials for maximal LFSRs can be found:  https://en.wikipedia.org/wiki/Linear-feedback_shift_register For example: ''z^13 + z^12 + z^11 + z^8 + 1''
  Sine Lookup : Lookup_n-D  NumberOfTableDimensions=1  BreakpointsForDimension1=[0:255]  IndexSearchMethod=Evenly spaced points  Table=sin([0:255]*2*pi/256)  InterpMethod=Flat  ExtrapMethod=Clip  DiagnosticForOutOfRangeInput=Error  UseLastTableValue=on  OutDataTypeStr=fixdt(1,16,14)  RndMeth=Simplest  InputSameDT=on
  awgn_imag : Outport
  awgn_real : Outport  Port=2
  wires:
  noise_std/1 -> Product3/2, Product2/2
  Product/1 -> Product3/1
  Product3/1 -> awgn_imag/1
  Cosine Lookup/1 -> Product1/1
  Random Number Generator/1(data) -> Cosine Lookup/1, Sine Lookup/1
  Random Number Generator1/1(data) -> Log Lookup/1
  Sine Lookup/1 -> Product/1
  Product1/1 -> Product2/1
  Constant/1 -> Random Number Generator/Enable, Random Number Generator1/Enable
  Constant1/1 -> Random Number Generator/1(reset), Random Number Generator1/1(reset)
  Log Lookup/1 -> Product/2, Product1/2
  Product2/1 -> awgn_real/1

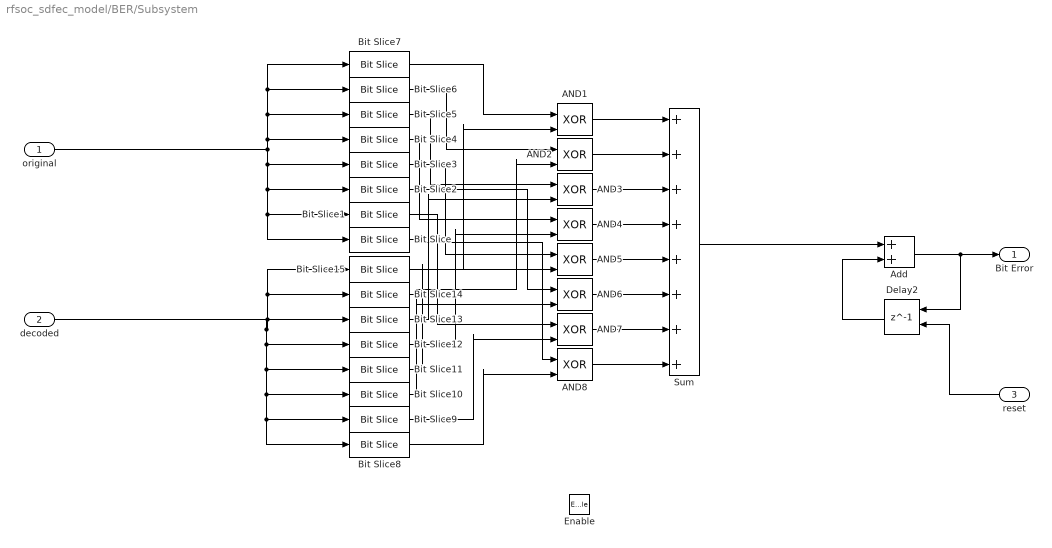
== system rfsoc_sdfec_model/BER/Subsystem ==
  original : Inport
  decoded : Inport  Port=2
  reset : Inport  Port=3
  Enable : EnablePort
  AND{1..8} (8 alike) : Logic  Operator=XOR  IconShape=distinctive  AllPortsSameDT=off  OutDataTypeStr=boolean
  Add : Sum  OutDataTypeStr=uint32
  Bit Slice : hdlsllib/Logic and Bit Operations/Bit Slice  lidx=0  ridx=0
      settings: SourceProductBaseCode=SL
  Bit Slice1 : hdlsllib/Logic and Bit Operations/Bit Slice  lidx=1  ridx=1
      settings: SourceProductBaseCode=SL
  Bit Slice10 : hdlsllib/Logic and Bit Operations/Bit Slice  lidx=2  ridx=2
      settings: SourceProductBaseCode=SL
  Bit Slice11 : hdlsllib/Logic and Bit Operations/Bit Slice  lidx=3  ridx=3
      settings: SourceProductBaseCode=SL
  Bit Slice12 : hdlsllib/Logic and Bit Operations/Bit Slice  lidx=4  ridx=4
      settings: SourceProductBaseCode=SL
  Bit Slice13 : hdlsllib/Logic and Bit Operations/Bit Slice  lidx=5  ridx=5
      settings: SourceProductBaseCode=SL
  Bit Slice14 : hdlsllib/Logic and Bit Operations/Bit Slice  lidx=6  ridx=6
      settings: SourceProductBaseCode=SL
  Bit Slice15 : hdlsllib/Logic and Bit Operations/Bit Slice  lidx=7  ridx=7
      settings: SourceProductBaseCode=SL
  Bit Slice2 : hdlsllib/Logic and Bit Operations/Bit Slice  lidx=2  ridx=2
      settings: SourceProductBaseCode=SL
  Bit Slice3 : hdlsllib/Logic and Bit Operations/Bit Slice  lidx=3  ridx=3
      settings: SourceProductBaseCode=SL
  Bit Slice4 : hdlsllib/Logic and Bit Operations/Bit Slice  lidx=4  ridx=4
      settings: SourceProductBaseCode=SL
  Bit Slice5 : hdlsllib/Logic and Bit Operations/Bit Slice  lidx=5  ridx=5
      settings: SourceProductBaseCode=SL
  Bit Slice6 : hdlsllib/Logic and Bit Operations/Bit Slice  lidx=6  ridx=6
      settings: SourceProductBaseCode=SL
  Bit Slice7 : hdlsllib/Logic and Bit Operations/Bit Slice  lidx=7  ridx=7
      settings: SourceProductBaseCode=SL
  Bit Slice8 : hdlsllib/Logic and Bit Operations/Bit Slice  lidx=0  ridx=0
      settings: SourceProductBaseCode=SL
  Bit Slice9 : hdlsllib/Logic and Bit Operations/Bit Slice  lidx=1  ridx=1
      settings: SourceProductBaseCode=SL
  Delay2 : Delay  DelayLength=1  ExternalReset=Level
      settings: InputPortMap=u0,r5
  Sum : Sum  Inputs=++++++++  OutDataTypeStr=fixdt(0,3,0)  SaturateOnIntegerOverflow=on
  Bit Error : Outport  InitialOutput=0
  wires:
  Bit Slice14/1 -> AND2/2
  original/1 -> Bit Slice/1, Bit Slice1/1, Bit Slice2/1, Bit Slice3/1, Bit Slice4/1, Bit Slice5/1, Bit Slice6/1, Bit Slice7/1
  AND5/1 -> Sum/5
  Delay2/1 -> Add/2
  Bit Slice15/1 -> AND1/2
  AND2/1 -> Sum/2
  Bit Slice6/1 -> AND2/1
  AND4/1 -> Sum/4
  decoded/1 -> Bit Slice8/1, Bit Slice9/1, Bit Slice10/1, Bit Slice11/1, Bit Slice12/1, Bit Slice13/1, Bit Slice15/1, Bit Slice14/1
  AND6/1 -> Sum/6
  Sum/1 -> Add/1
  AND7/1 -> Sum/7
  Bit Slice2/1 -> AND6/1
  AND8/1 -> Sum/8
  Bit Slice/1 -> AND8/1
  Bit Slice4/1 -> AND4/1
  Bit Slice3/1 -> AND5/1
  Bit Slice5/1 -> AND3/1
  Bit Slice7/1 -> AND1/1
  Bit Slice8/1 -> AND8/2
  Add/1 -> Bit Error/1, Delay2/1
  Bit Slice10/1 -> AND6/2
  Bit Slice12/1 -> AND4/2
  Bit Slice9/1 -> AND7/2
  Bit Slice1/1 -> AND7/1
  AND3/1 -> Sum/3
  Bit Slice13/1 -> AND3/2
  Bit Slice11/1 -> AND5/2
  AND1/1 -> Sum/1
  reset/1 -> Delay2/2

== system rfsoc_sdfec_model/Decode/Subsystem ==
  frame_out : Inport
  Enable : EnablePort
  LDPC Decoder : commblkcod2/LDPC Decoder  ParityCheckMat=parity_sparse  OutputFmt=Information part  DecisionType=Hard decision  OutputDataType=boolean  NumIter=64  DoParityCheck=on  OutputNumIter=off  OutputFinalChecks=off
      settings: SourceProductBaseCode=CM
  frame : Outport
  wires:
  frame_out/1 -> LDPC Decoder/1
  LDPC Decoder/1 -> frame/1

== system rfsoc_sdfec_model/Encoder/Encode ==
  frame_out : Inport
  Enable : EnablePort
  Cast To Boolean1 : DataTypeConversion  OutDataTypeStr=boolean
  Cast To Double : DataTypeConversion  OutDataTypeStr=double
  LDPC Encoder1 : commblkcod2/LDPC Encoder  ParityCheckMat=parity_sparse
      settings: SourceProductBaseCode=CM
  frame : Outport
  wires:
  LDPC Encoder1/1 -> Cast To Boolean1/1
  Cast To Boolean1/1 -> frame/1
  Cast To Double/1 -> LDPC Encoder1/1
  frame_out/1 -> Cast To Double/1

== system rfsoc_sdfec_model/QAM Mapping/QAM16 Generator ==
  bits : Inport
  Bit Concat1 : hdlsllib/Logic and Bit Operations/Bit Concat  numInputs=2
  Bit Slice1 : hdlsllib/Logic and Bit Operations/Bit Slice  lidx=1  ridx=0
      settings: SourceProductBaseCode=SL
  Bit Slice2 : hdlsllib/Logic and Bit Operations/Bit Slice  lidx=3  ridx=2
      settings: SourceProductBaseCode=SL
  Constant1 : Constant  Value=3  OutDataTypeStr=fixdt(1,4,0)  SampleTime=-1
  Constant2 : Constant  OutDataTypeStr=fixdt(1,4,0)  SampleTime=-1
  Constant3 : Constant  Value=-1  OutDataTypeStr=fixdt(1,4,0)  SampleTime=-1
  Constant4 : Constant  Value=-3  OutDataTypeStr=fixdt(1,4,0)  SampleTime=-1
  Multiport Switch : MultiPortSwitch  DataPortOrder=Zero-based contiguous  Inputs=4  zeroidx=on
  Multiport Switch1 : MultiPortSwitch  DataPortOrder=Zero-based contiguous  Inputs=4  zeroidx=on
  symbol : Outport
  wires:
  Multiport Switch/1 -> Bit Concat1/2  "I"
  Multiport Switch1/1 -> Bit Concat1/1  "Q"
  Bit Concat1/1 -> symbol/1
  Constant2/1 -> Multiport Switch1/3, Multiport Switch/5
  Constant1/1 -> Multiport Switch1/2, Multiport Switch/4
  Constant4/1 -> Multiport Switch1/4, Multiport Switch/2
  Constant3/1 -> Multiport Switch/3, Multiport Switch1/5
  bits/1 -> Bit Slice2/1, Bit Slice1/1
  Bit Slice2/1 -> Multiport Switch/1
  Bit Slice1/1 -> Multiport Switch1/1

== system rfsoc_sdfec_model/Random Number Generator/Random Number Generator ==
  reset : Inport
  enable : EnablePort
  bit0 : commseqgen3/PN Sequence Generator  poly='z^13 + z^12 + z^11 + z^8 + 1'  ini_sta=[ 1 1 0 0 1 1 1 0 0 0 1 1 0]  outBitMaskSource=Dialog parameter  shift=0  outVarSiz=off  maxOutSizeMode=Dialog parameter  maxOutSize=[10 1]  Ts=-1  sampPerFrame=1  reset=on  bitPackedOutputs=off  outDataType=boolean  numPackedBits=8  bitPackDataSigned=off  bitPackedOutDType=double
  bit1 : commseqgen3/PN Sequence Generator  poly='z^13 + z^12 + z^11 + z^8 + 1'  ini_sta=[ 1 0 0 1 0 0 1 1 1 0 1 0 0]  outBitMaskSource=Dialog parameter  shift=0  outVarSiz=off  maxOutSizeMode=Dialog parameter  maxOutSize=[10 1]  Ts=-1  sampPerFrame=1  reset=on  bitPackedOutputs=off  outDataType=boolean  numPackedBits=8  bitPackDataSigned=off  bitPackedOutDType=double
  bit2 : commseqgen3/PN Sequence Generator  poly='z^13 + z^12 + z^11 + z^8 + 1'  ini_sta=[ 0 0 1 0 1 1 1 0 1 1 0 1 1]  outBitMaskSource=Dialog parameter  shift=0  outVarSiz=off  maxOutSizeMode=Dialog parameter  maxOutSize=[10 1]  Ts=-1  sampPerFrame=1  reset=on  bitPackedOutputs=off  outDataType=boolean  numPackedBits=8  bitPackDataSigned=off  bitPackedOutDType=double
  bit3 : commseqgen3/PN Sequence Generator  poly='z^13 + z^12 + z^11 + z^8 + 1'  ini_sta=[ 0 0 1 1 1 1 0 1 0 1 1 1 0]  outBitMaskSource=Dialog parameter  shift=0  outVarSiz=off  maxOutSizeMode=Dialog parameter  maxOutSize=[10 1]  Ts=-1  sampPerFrame=1  reset=on  bitPackedOutputs=off  outDataType=boolean  numPackedBits=8  bitPackDataSigned=off  bitPackedOutDType=double
  bit4 : commseqgen3/PN Sequence Generator  poly='z^13 + z^12 + z^11 + z^8 + 1'  ini_sta=[ 1 1 1 0 0 0 1 0 1 1 1 1 0]  outBitMaskSource=Dialog parameter  shift=0  outVarSiz=off  maxOutSizeMode=Dialog parameter  maxOutSize=[10 1]  Ts=-1  sampPerFrame=1  reset=on  bitPackedOutputs=off  outDataType=boolean  numPackedBits=8  bitPackDataSigned=off  bitPackedOutDType=double
  bit5 : commseqgen3/PN Sequence Generator  poly='z^13 + z^12 + z^11 + z^8 + 1'  ini_sta=[ 0 0 0 0 0 1 1 1 0 1 0 1 1]  outBitMaskSource=Dialog parameter  shift=0  outVarSiz=off  maxOutSizeMode=Dialog parameter  maxOutSize=[10 1]  Ts=-1  sampPerFrame=1  reset=on  bitPackedOutputs=off  outDataType=boolean  numPackedBits=8  bitPackDataSigned=off  bitPackedOutDType=double
  bit6 : commseqgen3/PN Sequence Generator  poly='z^13 + z^12 + z^11 + z^8 + 1'  ini_sta=[ 0 1 1 1 1 1 0 1 0 1 1 0 1]  outBitMaskSource=Dialog parameter  shift=0  outVarSiz=off  maxOutSizeMode=Dialog parameter  maxOutSize=[10 1]  Ts=-1  sampPerFrame=1  reset=on  bitPackedOutputs=off  outDataType=boolean  numPackedBits=8  bitPackDataSigned=off  bitPackedOutDType=double
  bit7 : commseqgen3/PN Sequence Generator  poly='z^13 + z^12 + z^11 + z^8 + 1'  ini_sta=[ 0 0 1 0 1 0 1 1 0 0 0 0 0]  outBitMaskSource=Dialog parameter  shift=0  outVarSiz=off  maxOutSizeMode=Dialog parameter  maxOutSize=[10 1]  Ts=-1  sampPerFrame=1  reset=on  bitPackedOutputs=off  outDataType=boolean  numPackedBits=8  bitPackDataSigned=off  bitPackedOutDType=double
  concat : hdlsllib/Logic and Bit Operations/Bit Concat  numInputs=8
  data : Outport  InitialOutput=0
  wires:
  reset/1 -> bit0/1, bit1/1, bit2/1, bit3/1, bit4/1, bit5/1, bit6/1, bit7/1
  bit0/1 -> concat/1
  bit1/1 -> concat/2
  bit2/1 -> concat/3
  bit3/1 -> concat/4
  bit4/1 -> concat/5
  bit5/1 -> concat/6
  bit6/1 -> concat/7
  bit7/1 -> concat/8
  concat/1 -> data/1

== system rfsoc_sdfec_model/Random Number Generator/rising_edge ==
  in : Inport
  Data Type Conversion1 : DataTypeConversion  OutDataTypeStr=boolean  SaturateOnIntegerOverflow=on  RndMeth=Zero
  Delay15 : Delay  DelayLength=1  InitialCondition=1  InputProcessing=Columns as channels (frame based)
  Logical Operator2 : Logic  Operator=NOT  Inputs=1
  Logical Operator3 : Logic
  pulse : Outport
  wires:
  Logical Operator2/1 -> Logical Operator3/2
  in/1 -> Data Type Conversion1/1
  Data Type Conversion1/1 -> Logical Operator3/1, Delay15/1
  Logical Operator3/1 -> pulse/1
  Delay15/1 -> Logical Operator2/1

== system rfsoc_sdfec_model/Random Number Generator/tvalid hold ==
  en : Inport
  trigger : Inport  Port=2
  comparator : Inport  Port=3
  AND : Logic  IconShape=distinctive  AllPortsSameDT=off  OutDataTypeStr=boolean
  Delay2 : Delay  DelayLength=1
  Equal : RelationalOperator  OutDataTypeStr=boolean  RndMeth=Simplest
  HDL Counter : hdlsllib/Sources/HDL Counter  CountType=Free running  CountInit=0  CountStep=8  CountMax=25  CountFromType=Initial value  CountFrom=0  CountResetPort=on  CountLoadPort=off  CountEnbPort=on  CountDirPort=off  CountDataType=Unsigned  CountWordLen=32  CountFracLen=0  CountSampTime=1
  Multiport Switch : MultiPortSwitch  DataPortOrder=Zero-based contiguous  Inputs=2  zeroidx=on
  OR : Logic  Operator=OR  IconShape=distinctive  AllPortsSameDT=off  OutDataTypeStr=boolean
  enable : Outport
  wires:
  Multiport Switch/1 -> AND/2, enable/1, Delay2/1
  HDL Counter/1 -> Equal/1
  Equal/1 -> HDL Counter/1, OR/1
  trigger/1 -> Multiport Switch/3, OR/2
  comparator/1 -> Equal/2
  Delay2/1 -> Multiport Switch/2
  OR/1 -> Multiport Switch/1
  en/1 -> AND/1
  AND/1 -> HDL Counter/2

== system rfsoc_sdfec_model/Soft Demodulation/symmetric saturation ==
  soft_bits : Inport
  Bit Concat : hdlsllib/Logic and Bit Operations/Bit Concat  numInputs=3
  Bit Slice : hdlsllib/Logic and Bit Operations/Bit Slice  lidx=5  ridx=5
      settings: SourceProductBaseCode=SL
  Constant : Constant  Value=7.75  OutDataTypeStr=fixdt(1,6,2)  SampleTime=-1
  Constant2 : Constant  Value=-7.75  OutDataTypeStr=fixdt(1,6,2)  SampleTime=-1
  GreaterThan : RelationalOperator  Operator=>  OutDataTypeStr=boolean  RndMeth=Simplest
  GreaterThan1 : RelationalOperator  Operator=<  OutDataTypeStr=boolean  RndMeth=Simplest
  Multiport Switch : MultiPortSwitch  DataPortOrder=Zero-based contiguous  Inputs=2  zeroidx=on
  Multiport Switch1 : MultiPortSwitch  DataPortOrder=Zero-based contiguous  Inputs=2  zeroidx=on
  u : Outport
  wires:
  Bit Slice/1 -> Bit Concat/1, Bit Concat/2
  Multiport Switch1/1 -> Bit Concat/3, Bit Slice/1
  Bit Concat/1 -> u/1
  soft_bits/1 -> GreaterThan/1, Multiport Switch/2, GreaterThan1/1
  GreaterThan/1 -> Multiport Switch/1
  GreaterThan1/1 -> Multiport Switch1/1
  Multiport Switch/1 -> Multiport Switch1/2
  Constant/1 -> GreaterThan/2, Multiport Switch/3
  Constant2/1 -> GreaterThan1/2, Multiport Switch1/3
